simulink model "anndemo"  (Simulink 10.0)
settings: Solver=FixedStepDiscrete  StartTime=0.0  StopTime=1000  FixedStep=0.05  RelTol=1e-3  EnableMultiTasking=on
libraries: simulink3 x1, ann x1
settings Model: Creator=CAMPA  LastModifiedBy=unknown  ExtModeTrigMode=oneshot  ExtModeArmWhenConnect=off
settings DataIOCC: SignalLoggingSaveFormat=ModelDataLogs
settings OptimizationCC: BlockReduction=off  BooleanDataType=off  LifeSpan=auto
settings DebuggingCC: SaveWithParameterizedLinksMsg=none  SignalResolutionControl=TryResolveAllWithWarning  MultiTaskDSMMsg=warning  MultiTaskCondExecSysMsg=none  SFUnexpectedBacktrackingDiag=error  SFNoUnconditionalDefaultTransitionDiag=error  SFExecutionAtInitializationDiag=warning  ArithmeticOperatorsInVariantConditions=error
settings HardwareCC: ProdBitPerPointer=64  ProdBitPerSizeT=64  ProdBitPerPtrDiffT=64  ProdLargestAtomicFloat=Float  ProdIntDivRoundTo=Zero  ProdEndianess=LittleEndian  ProdWordSize=64  ProdHWDeviceType=Intel->x86-64 (Windows64)  TargetUnknown=on
settings SFSimCC: SimUseLocalCustomCode=on  CustomCodeUndefinedFunction=FilterOut
settings RTWCC: RTWUseLocalCustomCode=on
settings CodeAppCC: StateflowObjectComments=off
settings GRTTargetCC: TargetLangStandard=C99 (ISO)
settings ConfigComp: CovMetricSettings=dwe  CovHtmlReporting=off  CovSaveCumulativeToWorkspaceVar=off  CovSaveSingleToWorkspaceVar=off

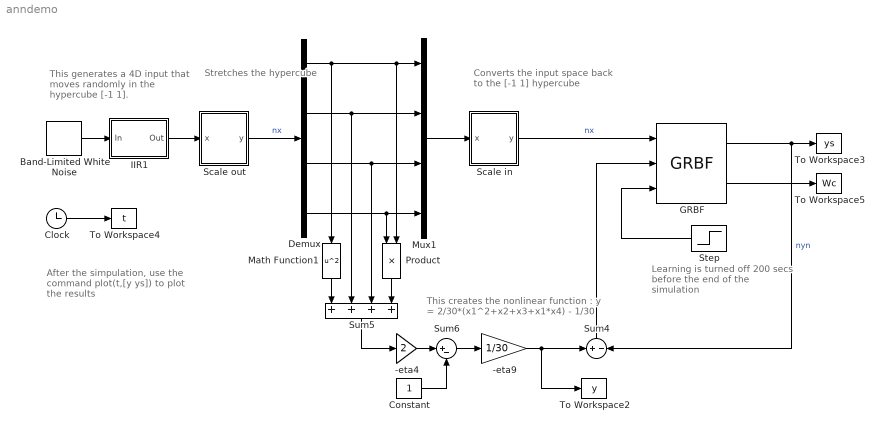
== system anndemo ==
  note: After the simpulation,
      | use the command
      | plot(t,[y ys])
      | to plot the results
  note: This generates a 4D input
      | that moves randomly in the
      | hypercube [-1 1].
  note: Stretches the
      | hypercube
  note: Converts the input
      | space back to the
      | [-1 1] hypercube
  note: This creates the nonlinear function :
      | y = 2/30*(x1^2+x2+x3+x1*x4) - 1/30
  note: Learning is turned off
      | 200 secs before the
      | end of the simulation
  -eta4 : Gain  Gain=2  SaturateOnIntegerOverflow=on  OutDataTypeStr=Inherit: Same as input  ParamDataTypeStr=Inherit: Same as input
  -eta9 : Gain  Gain=1/30  SaturateOnIntegerOverflow=on  OutDataTypeStr=Inherit: Same as input  ParamDataTypeStr=Inherit: Same as input
  Band-Limited White Noise : simulink3/Sources/Band-Limited White Noise  Cov=[1 1 1 1]  Ts=0.05  seed=1:4
      settings: SourceProductName=Simulink  SourceProductBaseCode=SL
  Clock : Clock
  Constant : Constant
  Demux : Demux
  GRBF : ann/GRBF  dim=[4 1]  nwrap="[100     1           10               1]"  eta=[1 1 1]*1e-3  gam=[1 1 1]*1e-6  lim=[1 1 1]*1e6  e1=0.2  e2="[0.3  0.2  0.999]"  e3=[0 0.5]  x0=zeros((4+2)*100+2,1)  T=0.05
  IIR1 : Subsystem  mask(Discrete Time First Order IIR){ni=4, a=0.25, x0=0, T=0.05}
      mask prompts: ni "Number of Channels"; a "Cutoff Frequency (a)"; x0 "Initial Condition"; T "Sample Time"
      mask help:
      | Each channel has the transfer function
      |   (1-exp(-aT))/(1-exp(-aT)(z^-1)) which is a good
      |   (pz-matched) approximation of a/(s+a) if 10*a*T<pi
      mask init:
      | A=[];B=[];C=[];D=[];
      | for i=1:ni,
      | A=[A,zeros(size(A,1),1);zeros(1,size(A,2)),exp(-a*T)];
      | B=[B,zeros(size(B,1),1);zeros(1,size(B,2)),1-exp(-a*T)];
      | C=[C,zeros(size(C,1),1);zeros(1,size(C,2)),exp(-a*T)];
      | D=[D,zeros(size(D,1),1);zeros(1,size(D,2)),1-exp(-a*T)];
      | end
      mask Help:
      | <p>
      |   Each channel has the transfer function
      |   (1-exp(-aT))/(1-exp(-aT)(z^-1)) which is a good
      |   (pz-matched) approximation of a/(s+a) if 10*a*T<pi
      | </p>
      mask Display: dpoly(a,[1 a],'s')
  Math Function1 : Math  Operator=square  SaturateOnIntegerOverflow=on
  Mux1 : Mux
  Product : Product  SaturateOnIntegerOverflow=on  RndMeth=Zero  InputSameDT=on  OutDataTypeStr=Inherit: Same as first input
  Scale in : Subsystem  mask(Scale){xmin=[0 -5 -6 -2], xmax=[1 0 6 7], ymin=[-1 -1 -1 -1], ymax=[1 1 1 1]}
      mask prompts: xmin "x min"; xmax "x max"; ymin "y min"; ymax "y max"
      mask help:
      | Scales the input vector x, ranging from xmin to xmax,
      |    to an output vector y, ranging from ymin to ymax
      mask Help:
      | Scales the input vector x, ranging from xmin to xmax,
      |    to an output vector y, ranging from ymin to ymax
  Scale out : Subsystem  mask(Scale){xmin=[-1 -1 -1 -1], xmax=[1 1 1 1], ymin=[0 -5 -6 -2], ymax=[1 0 6 7]}
      mask prompts: xmin "x min"; xmax "x max"; ymin "y min"; ymax "y max"
      mask help:
      | Scales the input vector x, ranging from xmin to xmax,
      |    to an output vector y, ranging from ymin to ymax
      mask Help:
      | Scales the input vector x, ranging from xmin to xmax,
      |    to an output vector y, ranging from ymin to ymax
  Step : Step  Time=800  Before=1  After=0  SampleTime=0.05
  Sum4 : Sum  Inputs=+|-  SaturateOnIntegerOverflow=on  InputSameDT=on  OutDataTypeStr=Inherit: Same as first input
  Sum5 : Sum  Inputs=++++  SaturateOnIntegerOverflow=on  InputSameDT=on  OutDataTypeStr=Inherit: Same as first input
  Sum6 : Sum  Inputs=|+-  SaturateOnIntegerOverflow=on  InputSameDT=on  OutDataTypeStr=Inherit: Same as first input
  To Workspace2 : ToWorkspace  VariableName=y  SampleTime=-1
  To Workspace3 : ToWorkspace  VariableName=ys  SampleTime=0.05
  To Workspace4 : ToWorkspace  VariableName=t  SampleTime=0.05
  To Workspace5 : ToWorkspace  VariableName=Wc  SampleTime=0.05
  wires:
  Demux/1 -> Math Function1/1, Product/2, Mux1/1
  Demux/2 -> Sum5/2, Mux1/2
  Demux/3 -> Sum5/3, Mux1/3
  Math Function1/1 -> Sum5/1
  Sum5/1 -> -eta4/1
  Mux1/1 -> Scale in/1(x)
  Constant/1 -> Sum6/2
  -eta4/1 -> Sum6/1
  Sum6/1 -> -eta9/1
  -eta9/1 -> Sum4/1, To Workspace2/1
  Product/1 -> Sum5/4
  Demux/4 -> Product/1, Mux1/4
  Band-Limited White Noise/1 -> IIR1/1(In)
  Scale out/1(y) -> Demux/1  "nx"
  Clock/1 -> To Workspace4/1
  IIR1/1(Out) -> Scale out/1(x)
  GRBF/1 -> To Workspace3/1, Sum4/2  "nyn"
  GRBF/2 -> To Workspace5/1
  Step/1 -> GRBF/3
  Scale in/1(y) -> GRBF/1  "nx"
  Sum4/1 -> GRBF/2

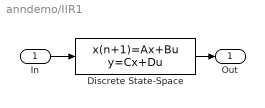
== system anndemo/IIR1 ==
  In : Inport
  Discrete State-Space : DiscreteStateSpace  A=A  B=B  C=C  D=D  InitialCondition=x0  SampleTime=T
  Out : Outport
  wires:
  Discrete State-Space/1 -> Out/1
  In/1 -> Discrete State-Space/1

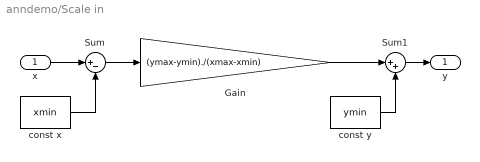
== system anndemo/Scale in ==
  x : Inport
  Gain : Gain  Gain=(ymax-ymin)./(xmax-xmin)  SaturateOnIntegerOverflow=on  OutDataTypeStr=Inherit: Same as input  ParamDataTypeStr=Inherit: Same as input
  Sum : Sum  Inputs=|+-  SaturateOnIntegerOverflow=on  InputSameDT=on  OutDataTypeStr=Inherit: Same as first input
  Sum1 : Sum  Inputs=|++  SaturateOnIntegerOverflow=on  InputSameDT=on  OutDataTypeStr=Inherit: Same as first input
  const x : Constant  Value=xmin
  const y : Constant  Value=ymin
  y : Outport
  wires:
  const y/1 -> Sum1/2
  Sum1/1 -> y/1
  Gain/1 -> Sum1/1
  const x/1 -> Sum/2
  Sum/1 -> Gain/1
  x/1 -> Sum/1

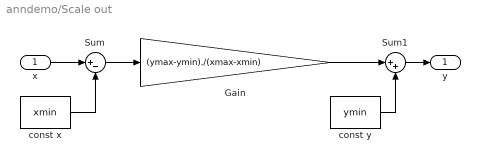
== system anndemo/Scale out ==
  x : Inport
  Gain : Gain  Gain=(ymax-ymin)./(xmax-xmin)  SaturateOnIntegerOverflow=on  OutDataTypeStr=Inherit: Same as input  ParamDataTypeStr=Inherit: Same as input
  Sum : Sum  Inputs=|+-  SaturateOnIntegerOverflow=on  InputSameDT=on  OutDataTypeStr=Inherit: Same as first input
  Sum1 : Sum  Inputs=|++  SaturateOnIntegerOverflow=on  InputSameDT=on  OutDataTypeStr=Inherit: Same as first input
  const x : Constant  Value=xmin
  const y : Constant  Value=ymin
  y : Outport
  wires:
  x/1 -> Sum/1
  Sum/1 -> Gain/1
  const x/1 -> Sum/2
  Gain/1 -> Sum1/1
  Sum1/1 -> y/1
  const y/1 -> Sum1/2
